simulink library "powerlib_extras"  (Simulink 6.0)
settings: Solver=ode45  SolverMode=SingleTasking  StartTime=0.0  StopTime=10.0  RelTol=1e-3
values from neighbouring files (symbols this model uses):
  Ts = get(handles.edit1,'string')    [powergui.m]
undefined symbols (not defined in the file or in its folder): Ac, Bc, Cc, Dc, Delay_discrete, dend, DiscIntNeverNeededParam, extra_sc, j, numd, test_alpha
libraries: powerlib2 x112, powerlib_extras x70, simulink_extras x25, simulink x12, powerlib_models x8
(part 1 of 9)
Description:
  | Powerlib_extras library for the Power System Blockset 2.1
settings Model: RequirementInfo=9  Creator=patrice  LastModifiedBy=batserve  ModifiedHistory=New version of the Timer block of the control library  ExtModeAutoUpdateStatusClock=off
settings DataIOCC: SignalLoggingName=logsOut
settings OptimizationCC: BooleanDataType=off
settings DebuggingCC: CheckExecutionContextPreStartOutputMsg=on  CheckExecutionContextRuntimeOutputMsg=on  SolverPrmCheckMsg=none
settings HardwareCC: TargetUnknown=on

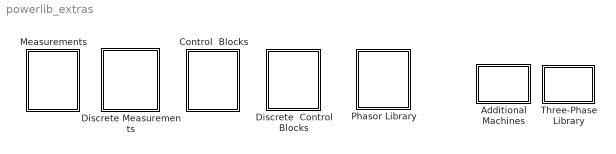
== system powerlib_extras ==
  Additional Machines : Subsystem
      mask Display: disp('obsolete\nblocks')
  Control  Blocks : Subsystem
  Discrete Measurements : Subsystem
  Discrete  Control Blocks : Subsystem
  Measurements : Subsystem
  Phasor Library : Subsystem
  Three-Phase Library : Subsystem
      mask Display: disp('Obsolete\nblocks')

== system powerlib_extras/Additional Machines ==
  DC Machine : powerlib2/Machines/DC Machine  RLa="[ 0.6  0.012]"  RLf="[ 240  120]"  Laf=1.8  J=1  Bm=0  Tf=0  w0=1  PSBOutputType=110
  Discrete DC_Machine : Subsystem  mask(Discrete DC machine){RLa=[0.5  0.01], RLf=[240  0], Laf=1.23, J=0.05, Bm=0.02, Tf=0, w0=0, PSBOutputType=110, Ts=50e-6}
      mask prompts: RLa "Armature resistance and inductance [Ra (ohms) La (H) ]"; RLf "Field resistance and inductance [Rf (ohms) Lf (H) ]"; Laf "Field-armature mutual inductance Laf (H) :"; J "Total inertia J (kg.m^2)"; Bm "Viscous friction coefficient Bm (N.m.s)"; Tf "Coulomb friction torque Tf (N.m)"; w0 "Initial speed (rad/s) :"; PSBOutputType "Output type"; Ts "Sample time (s) :"
      mask help:
      | This discrete block implements a separately excited DC machine. Access is provided  to the field connections so that the machine can be used as a shunt-connected or a series-connected  DC machine.
      |
      | Input 1 and output 1 : positive and negative armature terminals
      | Input 2 and output 2 : positive and negative field terminals
      | Input 3    : Load torque
      | Output 3 : Simulink measurement output [ w Ia If Te ]
      mask init:
      | Ra=RLa(1); La=RLa(2);
      | Rf=RLf(1); Lf=RLf(2);
      mask Help:
      | This block implements a separately excited DC machine. Access is provided  to the field connections so that the machine can be used as a shunt-connected or a series-connected  DC machine.
      | 
      | <pre>
      | The model implements the following electrical and mechanical equations:
      |     Vf  = (Rf+sLf )*If
      |     Va =   (w*Laf)*If  +  (Ra+sLaa)*Ia
      |     Te = Laf*If*Ia
      |     Te = J*dw/dt + Bm*w+ Tf + TL
      | where:
      |     Va, Vf = Armature anf field voltages (V)
      |     Ia , If = Armature anf field currents (A)
      |     w = Rotor speed (rad/s)
      |     s = Laplace derivation operator = d/dt
      |     Te = Electrical torque (N.m)
      |     TL = Load torque (N.m)
      |     Tv = Bm*w= Viscous friction torque (N.m)
      |     Tf = Coulomb friction torque (N.m)
      | 
      | Input 1 and output 1 : positive and negative armature terminals
      | Input 2 and output 2 : positive and negative field terminals
      | Input 3 : Load torque
      | Output 3 : Simulink measurement output [ w Ia If Te ]
      | 
      | In motor mode the Load torque applied on the shaft should be positive.
      | </pre>
      mask Display: plot(-80,-80,80,80,[0,9,18,24,29,30,29,24,18,9,0,-9,-18,-24,-29,-30,-29,-24,-18,-9,0],[30,29,24,18,9,0,-9,-18,-24,-29,-30,-29,-24,-18,-9,0,9,18,24,29,30],[-29,-35,-35,-29],[-8,-8,8,8],[29,35,35,29],[-8,-8,8,8],[-35,-55],[0,0],[35,55],[0,0],[-78,-50,-50,-49,-45,-39,-33,-26,-21,-18,-17,-19,-22,-22,-26,-27,-25,-22,-16,-9,-3,2,6,6,4,1,1,-3,-4,-2,2,7,14,20,26,29,30,28,24,24,21,20,21,25,31,37,44,49,50,50,50,78]*.7,[58,58,57.2,49.2,42.8,38.8,38,39.6,44.4,51.6,59.6,67.6,72.4,72.4,65.2,57.2,49.2,42.8,38.8,38,39.6,44.4,51.6,59.6,67.6,72.4,72.4,65.2,57.2,49.2,42.8,38.8,38,39.6,44.4,51.6,59.6,67.6,72.4,72.4,65.2,57.2,49.2,42.8,38.8,38,39.6,44.4,51.6,58,58,58]*.6+15 );

== system powerlib_extras/Control  Blocks ==
  note: __________ Filters__________
  note: _____________ Pulse Generators_____________
  note: __Phase-Locked Loop (PLL) Systems _______
  note: ___________________________ Miscellaneous_____________________________
  note: ___Signal Generators____
  " Synchronized 12-Pulse Generator" : Subsystem  mask(Synchronized 12-pulse generator){freq=60, pwidth=35, Double_Pulse=on}
      mask prompts: freq "Frequency of synchronisation voltages (Hz) :"; pwidth "Pulse width (degrees) :"; Double_Pulse "Double pulsing"
      mask help:
      | Use this block to fire the 12 thyristors of a 12-pulse converter. Outputs PY and PD are two vectors of 6 pulses (0-1) to be sent to the two 6-pulse half bridges connected respectively to the Wye(Y) and Delta (D) connected windings of the YYD (Delta Lagging)  converter transformer.
      |
      | Pulses are individually synchronized on the 6 commutation voltages and generated alpha degrees after the increasing zero-crossings of the commutation voltages. The D pulses are lagging the Y pulses by  30 degrees.
      |
      | When the 'Douple pulsing' option is checked, two pulses are sent to each thyristor: a 1st pulse when the aplha angle is reached, then a 2nd pulse 60 degrees later, when the next thyristor is fired.
      mask Help: web(psbhelp)
      mask Display: plot(0,0,100,100,[80 62 62 47 47 30],[40 40 60 60 40 40]-5)
  1-phase  PLL : Subsystem  mask(1-phase PLL){Par_Init=[0 60], ParK=[120 2800]}
      mask prompts: Par_Init "Initial inputs:[ Phase(degrees)   Frequency(Hz) ]"; ParK "Regulator gains [ Kp  Ki ]"
      mask help:
      | This Phase Locked Loop (PLL) system can be used  to synchronize on a variable frequency sinusoidal signal.
      |
      | Input 1: Normalized input signal V(pu)
      |
      | Output 1:  Measured frequency (Hz) = w/(2pi)
      | Output 2:  Ramp w.t  varying between  0 and 2*pi, synchronized on the zero-crossing (rising) of  the input signal
      | Output 3: Vector [sin(wt) cos(wt)]
      mask init:
      | Kp=ParK(1);
      | Ki=ParK(2);
      | Phase_Init=Par_Init(1);
      | Finit=Par_Init(2);
  1st-Order  Filter : Subsystem  mask(First-Order Filter){FilterType=Lowpass, Tc=12e-3, Initialize=off, Vac_Init=[0.8 -25 60], Vdc_Init=-0.4, PlotResponse=off, param1=[1 500 1]}
      mask prompts: FilterType "Filter Type:"; Tc "Time constant (s):"; Initialize "Initialize filter states"; Vac_Init "AC initial input: [ Mag  Phase(degrees)  Freq(Hz) ]"; Vdc_Init "DC Initial input:"; PlotResponse "Plot filter response"; param1 "Frequency range(Hz) : [Start  End  Inc.]"
      mask init:
      | switch FilterType
      | case 1, % Lowpass
      |        X=[0 1 2 3 4];
      |        Y=[-2 -2 -3 -4 -4];
      |        numc=1;
      |        denc=[Tc 1];
      |  case 2,   % Highpass
      |        X=[0 1 2 3 4];
      |        Y=[-4 -4 -3 -2 -2];
      |         numc=[1 0];
      |         denc=[1 1/Tc];
      | end
      | %
      | [Ac,Bc,Cc,Dc]=tf2ss(numc,denc);
      | %
      | %
      | if Initialize==1  % Compute initial conditions on states
      | u1=Vac_Init(1)*exp(j*Vac_Init(2)*pi/180);
      | u2=Vdc_Init*exp(j*90*pi/180);
      | u=u1+u2;
      | u0=imag(u); % input at  t=0;
      | I=eye(size(Ac));
      | sI1=I*j*(2*pi*Vac_Init(3));
      | sI2=I*j*0;
      | x=inv(sI1-Ac)*Bc*u1 + inv(sI2-Ac)*Bc*u2;
      | x0c=imag(x);
      | else
      | x0c=0;
      | end
      | %
      | if PlotResponse==1 % Plot frequency and step response
      | t=[0:Tc/1000:7*Tc];
      | f=param1(1):param1(3):param1(2);
      | w=2*pi*f;
      | switch FilterType
      | 	case 1, % Lowpass
      | 		Ystep=1 - exp(-t/Tc);
      | 		RepFreq=1./(1+Tc*j.*w);
      | 	case 2,   % Highpass
      | 		Ystep=exp(-t/Tc);
      | 		RepFreq=1./(1 + (1./(Tc*j.*w)));
      | end
      | %
      | Mag=abs(RepFreq);
      | Pha=angle(RepFreq)*180/pi;
      | %
      | figure(1)
      | subplot(2,1,1)
      | plot(f,Mag)
      | grid
      | title('Bode Diagram')
      | ylabel('Magnitude')
      | subplot(2,1,2)
      | plot(f,Pha)
      | ylabel('Phase (deg)')
      | xlabel('Frequency (Hz)')
      | grid
      | figure(2)
      | plot(t,Ystep)
      | grid
      | ylabel('Amplitude')
      | xlabel('Time (s)')
      | title('Step Response')
      | end
      mask StyleString: popup(Lowpass|Highpass),edit,checkbox,edit,edit,checkbox,edit
      mask CallbackString: ||parametres=get_param(gcb,'MaskValues');p3=parametres{3};p6=parametres{6};if strcmp(p3,'on');param4='on';param5='on';else;param4='off';param5='off';end;if strcmp(p6,'on');param7='on';else;param7='off';end;visible={'on','on','on',param4,param5,'on',param7};set_param(gcb,'MaskVisibilities',visible)|||parametres=get_param(gcb,'MaskValues');p3=parametres{3};p6=parametres{6};if strcmp(p3,'on');param4='on';param5='on';else;param4='off';param5='off';end;if strcmp(p6,'on');param7='on';else;param7='off';end;visible={'on','on','on',param4,param5,'on',param7};set_param(gcb,'MaskVisibilities',visible)|
      mask Display: plot(X,Y);
  2nd-Order Filter : Subsystem  mask(2nd-Order Filter){FilterType=Lowpass, Fo=200, Zeta=0.707, Initialize=off, Vac_Init=[1 45 60], Vdc_Init=-0.5, PlotResponse=off, param1=[1 500 1]}
      mask prompts: FilterType "Filter Type:"; Fo "Cut-off frequency (Hz):"; Zeta "Damping factor Zeta ( Q = 1 / (2*Zeta) ):"; Initialize "Initialize filter states"; Vac_Init "AC initial input: [ Mag  Phase(degrees)  Freq(Hz) ]"; Vdc_Init "DC Initial input:"; PlotResponse "Plot filter response"; param1 "Frequency range(Hz) : [Start  End  Inc.]"
      mask init:
      | Wo=2*pi*Fo;
      | str=sprintf(' Fo=%iHz\n\n',Fo);
      | switch FilterType
      | case 1, % Lowpass
      |        X=[0 1 2 3 4];
      |        Y=[-2 -2 -3 -4 -4];
      |        n2=0;n1=0;n0=Wo*Wo;
      |        d2=1;d1=2*Zeta*Wo;d0=Wo*Wo;
      |  case 2,   % Highpass
      |        X=[0 1 2 3 4];
      |        Y=[-4 -4 -3 -2 -2];
      |        n2=1;n1=0;n0=0;
      |        d2=1;d1=2*Zeta*Wo;d0=Wo*Wo;
      |     case 3,   % Bandpass
      |        X=[0 1 2 3 4 5 ];
      |        Y=[-3 -3 -2 -2 -3 -3];
      |        n2=0;n1=2*Zeta*Wo;n0=0;
      |        d2=1;d1=2*Zeta*Wo;d0=Wo*Wo;
      |     case 4,  %Bandstop (Notch)
      |        X=[0 1 2 3 4 5 ];
      |        Y=[-2 -2 -3 -3 -2 -2];
      |        n2=1;n1=0;n0=Wo*Wo;
      |        d2=1;d1=2*Zeta*Wo;d0=Wo*Wo;
      |     end
      | %
      | numc=[n2 n1 n0];
      | denc=[d2 d1 d0];
      | [Ac,Bc,Cc,Dc]=tf2ss(numc,denc);
      | %
      | if Initialize==1  % Compute initial conditions on states
      | u1=Vac_Init(1)*exp(j*Vac_Init(2)*pi/180);
      | u2=Vdc_Init*exp(j*90*pi/180);
      | u=u1+u2;
      | u0=imag(u); % input at  t=0;
      | I=eye(size(Ac));
      | sI1=I*j*(2*pi*Vac_Init(3));
      | sI2=I*j*0;
      | x=inv(sI1-Ac)*Bc*u1 + inv(sI2-Ac)*Bc*u2;
      | x0c=imag(x);
      | else
      | x0c=0;
      | end
      | %
      | if PlotResponse==1 % Plot frequency and step response
      | if Zeta==1
      | 	z=1+1e-12;
      | else
      | 	z=Zeta;
      | end
      | wn=Wo;
      | t=[0:1/(z*wn)/1000:7/(z*wn)];
      | f=param1(1):param1(3):param1(2);
      | w=2*pi*f;
      | switch FilterType
      | 	case 1, % Lowpass
      | 		Ystep=wn^2*(1/wn^2+1/(4*z^2*wn^2-4*wn^2)^(1/2)*(1/(-z*wn+1/2*(4*z^2*wn^2-4*wn^2)^(1/2))*exp((-z*wn+1/2*(4*z^2*wn^2-4*wn^2)^(1/2))*t)-1/(-z*wn-1/2*(4*z^2*wn^2-4*wn^2)^(1/2))*exp((-z*wn-1/2*(4*z^2*wn^2-4*wn^2)^(1/2))*t)));
      | 		numFreq=wn^2;
      | 	case 2,   % Highpass
      | 		Ystep=-exp(-z*wn*t)/(z-1)/(z+1).*cos((-wn^2*(z-1)*(z+1))^(1/2)*t)+exp(-z*wn*t)/(z-1)/(z+1)*z^2.*cos((-wn^2*(z-1)*(z+1))^(1/2)*t)+z/wn*exp(-z*wn*t)/(z-1)/(z+1)*(wn^2-z^2*wn^2)^(1/2).*sin((-wn^2*(z-1)*(z+1))^(1/2)*t);
      | 		numFreq=-w.^2;
      | 	case 3,   % Bandpass
      | 		Ystep=2*z*wn/(4*z^2*wn^2-4*wn^2)^(1/2)*(exp((-z*wn+1/2*(4*z^2*wn^2-4*wn^2)^(1/2))*t)-exp((-z*wn-1/2*(4*z^2*wn^2-4*wn^2)^(1/2))*t));
      | 		numFreq=2*Zeta*wn.*w*j;
      | 	case 4,  %Bandstop (Notch)
      | 		Ystep=1+2*z/wn*exp(-z*wn*t)/(z-1)/(z+1)*(wn^2-z^2*wn^2)^(1/2).*sin((-wn^2*(z-1)*(z+1))^(1/2)*t);	
      | 		numFreq=wn^2-w.^2;
      | end
      | %
      | denFreq=(wn^2-w.^2) + 2*Zeta*wn*j.*w;
      | RepFreq=numFreq./denFreq;
      | Mag=abs(RepFreq);
      | Pha=angle(RepFreq)*180/pi;
      | %
      | figure(1)
      | subplot(2,1,1)
      | plot(f,Mag)
      | grid
      | title('Bode Diagram')
      | ylabel('Magnitude')
      | subplot(2,1,2)
      | plot(f,Pha)
      | ylabel('Phase (deg)')
      | xlabel('Frequency (Hz)')
      | grid
      | figure(2)
      | plot(t,real(Ystep))
      | grid
      | ylabel('Amplitude')
      | xlabel('Time (s)')
      | title('Step Response')
      | end
      mask StyleString: popup(Lowpass|Highpass|Bandpass|Bandstop (Notch)),edit,edit,checkbox,edit,edit,checkbox,edit
      mask CallbackString: |||parametres=get_param(gcb,'MaskValues');p4=parametres{4};p7=parametres{7};if strcmp(p4,'on');param5='on';param6='on';else;param5='off';param6='off';end;if strcmp(p7,'on');param8='on';else;param8='off';end;visible={'on','on','on','on',param5,param6,'on',param8};set_param(gcb,'MaskVisibilities',visible)|||parametres=get_param(gcb,'MaskValues');p4=parametres{4};p7=parametres{7};if strcmp(p4,'on');param5='on';param6='on';else;param5='off';param6='off';end;if strcmp(p7,'on');param8='on';else;param8='off';end;visible={'on','on','on','on',param5,param6,'on',param8};set_param(gcb,'MaskVisibilities',visible)|
      mask Display:
      | plot(X,Y);
      | disp(str);
  3-phase  Programmable Source : Subsystem  mask(3-phase Programmable Source){Par_Vps=[1.0 -20  60], VariationEntity=Amplitude, VariationType=Step, VariationStep=-0.5, VariationRate=10, VariationMag=0.3, VariationFreq=2, Par_Timing_Variation=[0.1 1.2], SinglePhase=off, Yampli=[1 0.8 1.2 1.0], Xtime=[0 0.1 0.15 0.2], HarmonicGeneration=off, Par_HarmoA=[3 0.2 -25 0], Par_HarmoB=[2 0.15 35 2], Par_Timing_Harmo=[0.05  3]}
      mask prompts: Par_Vps "Positive-sequence: [ Amplitude  Phase(degrees)   Freq. (Hz) ]"; VariationEntity "Time variation of:"; VariationType "Type of variation:"; VariationStep "Step magnitude:"; VariationRate "Rate of change (value/s):"; VariationMag "Amplitude of the modulation:"; VariationFreq "Frequency of the modulation(Hz):"; Par_Timing_Variation "Variation timing (s) : [ Start   End ]"; SinglePhase "1-phase only"; Yampli "Amplitude values:"; Xtime "Time values:"; HarmonicGeneration "Harmonic generation:"; Par_HarmoA "A:  [ Order(n)   Amplitude  Phase(degrees)  Seq(0, 1 or 2) ]"; Par_HarmoB "B:  [ Order(n)   Amplitude  Phase(degrees)  Seq(0, 1 or 2) ]"; Par_Timing_Harmo "Harmonic timing (s) : [ Start   End ]"
      mask help: Use this block to generate a set of three-phase sinusoidal voltages or currents a, b and c. Time variation for the amplitude, phase and frequency of the fundamental can be pre-programmed. In addition, two harmonics can be surimposed on the fundamental.
      mask init:
      | Mag_Vps=Par_Vps(1);
      | Phase_Vps=Par_Vps(2);
      | Freq_Vps=Par_Vps(3);
      | 
      | Ton_Variation=Par_Timing_Variation(1);
      | Toff_Variation=Par_Timing_Variation(2);
      | n_HarmoA=Par_HarmoA(1);
      | Mag_HarmoA=Par_HarmoA(2);
      | Phase_HarmoA=Par_HarmoA(3);
      | Seq_HarmoA=Par_HarmoA(4);
      | if n_HarmoA==0
      |     Phase_HarmoA=90;
      |     Seq_HarmoA=0;
      | end
      | n_HarmoB=Par_HarmoB(1);
      | Mag_HarmoB=Par_HarmoB(2);
      | Phase_HarmoB=Par_HarmoB(3);
      | Seq_HarmoB=Par_HarmoB(4);
      | if n_HarmoB==0
      |     Phase_HarmoB=90;
      |     Seq_HarmoB=0;
      | end
      | Ton_Harmo=Par_Timing_Harmo(1);
      | Toff_Harmo=Par_Timing_Harmo(2);
      | 
      | if Xtime(1)~=0,
      | Xtime=[0 Xtime];
      | Yampli=[0 Yampli];
      | end
      | n=length(Xtime); vec_dt= [Xtime,0] - [0,Xtime] ; vec_dt=vec_dt(2:n);
      mask StyleString: edit,popup(None|Amplitude|Phase|Frequency),popup(Step|Ramp|Modulation|Table of time-amplitude pairs),edit,edit,edit,edit,edit,checkbox,edit,edit,checkbox,edit,edit,edit
      mask CallbackString: |parametres=get_param(gcb,'MaskValues');p2=parametres{2};p3=parametres{3};p12=parametres{12};if strcmp(p3,'Step');param4='on';param5='off';param6='off';param7='off';param8='on';param9='off';param10='off';param11='off';elseif strcmp(p3,'Ramp');param4='off';param5='on';param6='off';param7='off';param8='on';param9='off';param10='off';param11='off';elseif strcmp(p3,'Modulation');param4='off';param5='off';param6='on';param7='on';param8='on';param9='off';param10='off';param11='off';else;param4='off';param5='off';param6='off';param7='off';param8='off';param9='on';param10='on';param11='on';end;if strcmp(p2,'None');param3='off';param4='off';param5='off';param6='off';param7='off';param8='off';param9='off';param10='off';param11='off';else;param3='on';end;if strcmp(p12,'on');param13='on';param14='on';param15='on';else;param13='off';param14='off';param15='off';end;visible={'on','on',param3,param4,param5,param6,param7,param8,param9,param10,param11,'on',param13,param14,param15};set_param(gcb,'MaskVisibilities',visible)|parametres=get_param(gcb,'MaskValues');p2=parametres{2};p3=parametres{3};p12=parametres{12};if strcmp(p3,'Step');param4='on';param5='off';param6='off';param7='off';param8='on';param9='off';param10='off';param11='off';elseif strcmp(p3,'Ramp');param4='off';param5='on';param6='off';param7='off';param8='on';param9='off';param10='off';param11='off';elseif strcmp(p3,'Modulation');param4='off';param5='off';param6='on';param7='on';param8='on';param9='off';param10='off';param11='off';else;param4='off';param5='off';param6='off';param7='off';param8='off';param9='on';param10='on';param11='on';end;if strcmp(p2,'None');param3='off';param4='off';param5='off';param6='off';param7='off';param8='off';param9='off';param10='off';param11='off';else;param3='on';end;if strcmp(p12,'on');param13='on';param14='on';param15='on';else;param13='off';param14='off';param15='off';end;visible={'on','on',param3,param4,param5,param6,param7,param8,param9,param10,param11,'on',param13,param14,param15};set_param(gcb,'MaskVisibilities',visible)|||||||||parametres=get_param(gcb,'MaskValues');p2=parametres{2};p3=parametres{3};p12=parametres{12};if strcmp(p3,'Step');param4='on';param5='off';param6='off';param7='off';param8='on';param9='off';param10='off';param11='off';elseif strcmp(p3,'Ramp');param4='off';param5='on';param6='off';param7='off';param8='on';param9='off';param10='off';param11='off';elseif strcmp(p3,'Modulation');param4='off';param5='off';param6='on';param7='on';param8='on';param9='off';param10='off';param11='off';else;param4='off';param5='off';param6='off';param7='off';param8='off';param9='on';param10='on';param11='on';end;if strcmp(p2,'None');param3='off';param4='off';param5='off';param6='off';param7='off';param8='off';param9='off';param10='off';param11='off';else;param3='on';end;if strcmp(p12,'on');param13='on';param14='on';param15='on';else;param13='off';param14='off';param15='off';end;visible={'on','on',param3,param4,param5,param6,param7,param8,param9,param10,param11,'on',param13,param14,param15};set_param(gcb,'MaskVisibilities',visible)|||
  3-phase PLL : Subsystem  mask(3-phase PLL){Par_Init=[0 60], ParK=[60 1400]}
      mask prompts: Par_Init "Initial inputs:[ Phase(degrees)   Frequency(Hz) ]"; ParK "Regulator gains [ Kp  Ki ]"
      mask help:
      | This Phase Locked Loop (PLL) system can be used  to synchronize on a set of variable frequency, three-phase sinusoidal signals.
      |
      | Input 1: Vector containing the normalized
      |              three-phase signals [Va Vb Vc]
      | Output 1:  Measured frequency (Hz) = w/(2pi)
      | Output 2:  Ramp w.t   varying between  0 and 2*pi,
      | synchronized on zero crossings of the fundamental (positive-sequence) of phase A.
      | Output 3: Vector [sin(wt) cos(wt)]
      mask init:
      | Kp=ParK(1);
      | Ki=ParK(2);
      | Phase_Init=Par_Init(1);
      | Finit=Par_Init(2);
  Bistable : Subsystem  AncestorBlock=|  mask(Bistable Flip-Flop (Priority to Set or Reset)){priority=Set, ic=0}
      | powerlib_extras/Discrete 
      | Control Blocks/Discrete
      | Bistable
      mask prompts: priority "Priority to input:"; ic "Initial Q output (0/1):"
      mask help:
      | SR Flip-Flop block, with priority given either  to the Set  (S) or Reset  (R) input.
      |
      | Priority to Set: If inputs S (set) and R (reset) are TRUE (1) simultaneously, the output Q is set to TRUE (1).
      |
      | Priority to Reset: If inputs S (set) and R (reset) are TRUE (1) simultaneously, the output Q is reset to FALSE (0).
      |
      | The  Q! output  is the complement of the Q output.
      | The initial value of the Q output  is specified by the parameter "Initial Q output".
      mask init:
      | if (priority==1)   % RESET
      |  str1 = '[R]';
      |  str2 = 'S';
      | else
      | str1= 'R';
      | str2 = '[S]';
      | end
      mask StyleString: popup(Reset|Set),edit
      mask Display:
      | plot(0,0,100,100);
      | text(5,25,str1);
      | text(5,75,str2);
      | text(72,25,'!Q');
      | text(78,75,'Q');
  Edge Detector : Subsystem  mask(Edge Detector){model=Rising, ic=0}
      mask prompts: model "Edge:"; ic "Input at t = -eps:"
      mask help:
      | This block compares its present input to its previous input.
      |
      | If the input  is a logic signal (TRUE (1) or FALSE (0), the output is a one-step boolean signal TRUE  when  the specified edge (Rising, Falling or Either)  is detected.
      |
      | This block can also be used to detect the slope polarity of a continuous signal. For example, if the specified edge is  "Rising", the output is TRUE as long as the slope of the input signal is positive.
      |
      | The input value at time preceeding t=0 is specified by the parameter "Input at t=-eps"
      mask init:
      | if model~=3,
      | 	x1 = (model -1)*20;
      |     x2 = (model -1)*60;
      | 	X1=[5,20,20,35]+25; Y1=[20+x2,20+x2,80-x2,80-x2];
      | 	X2=[5,20,35]+25;    Y2=[40+x1,60-x1,40+x1];
      | 	X3=[];X4=[];Y3=[];Y4=[];
      | else
      | 	x1 = 20;
      | 	x2 = 60;
      | 	X1=[5,20,20,35]+8; Y1=[20,20,80,80];
      | 	X2=[5,20,35]+8;    Y2=[40,60,40];
      | 	X3=[5,20,20,35]+53; Y3=[20+x2,20+x2,80-x2,80-x2];
      | 	X4=[5,20,35]+53;    Y4=[40+x1,60-x1,40+x1];
      | end
      mask StyleString: popup(Rising|Falling|Either),edit
      mask Display: plot(0,0,100,100, X1,Y1,X2,Y2,X3,Y3,X4,Y4);
  Monostable : Subsystem  mask(Monostable Flip-Flop){EdgeDetect=Either, t_mono=0.015, ic=0}
      mask prompts: EdgeDetect "Edge detection"; t_mono "Pulse duration (s):"; ic "Input at t = -eps:"
      mask help:
      | After being triggered  by the specified edge (Rising, Falling or Either), this block outputs a pulse (TRUE signal) for the time specified by parameter "Pulse duration".
      | If the specified edge is detected while the output is TRUE, the monostable is not retriggered
      |
      | The input value (0/1) at time preceeding t = 0 is specified by the parameter "input at t = -eps".
      mask init:
      | str=sprintf('%g %c',t_mono,'s');
      | if (EdgeDetect ~=3)
      |     x1 = (EdgeDetect -1)*10;
      |     x2 = (EdgeDetect -1)*30;
      | 	X1=[15-8,25,25,35+8]+0; Y1=[65+x2,65+x2,95-x2,95-x2];
      | 	X2=[15,25,35]+0;   Y2=[75+x1,85-x1,75+x1];
      | 	X3=[];X4=[];Y3=[];Y4=[];	
      | else
      | 	x1 = 10;
      | 	x2 = 30;
      | 	X1=[15,25,25,35]-14;  Y1=[65,65,95,95];
      | 	X2=[15,25,35]-14;    Y2=[75,85,75];
      | 	X3=[15,25,25,35]+14; Y3=[65+x2,65+x2,95-x2,95-x2];
      | 	X4=[15,25,35]+14;   Y4=[75+x1,85-x1,75+x1];
      | end
      mask StyleString: popup(Rising|Falling|Either),edit,edit
      mask Display:
      | plot(0,0,100,100,[100 75 75 25 25 0],[25 25 50 50 25 25]-0,X1,Y1,X2,Y2,X3,Y3,X4,Y4);
      | text(45,37,'T');
      | text(15,15,str);
  On/Off Delay : Subsystem  AncestorBlock=|  mask(On/Off Delay ){type_delay=On delay, delay=0.01, ic=0}
      | powerlib_extras/Discrete 
      | Control Blocks/Discrete
      | On//Off Delay
      mask prompts: type_delay "Type:"; delay "Time delay:"; ic "Input at t = -eps (0/1):"
      mask help:
      | Apply a delay on the input signal when the input changes to TRUE (1) or FALSE (0).
      |
      | On delay: When the input becomes TRUE, the output becomes TRUE after the specified time delay as long as the input is still TRUE. If the input becomes FALSE before the time delay has expired , the output stays FALSE.
      |
      | Off delay: When the input becomes FALSE, the output becomes FALSE after the specified time delay as long as the input is still FALSE. If the input becomes TRUE before the time delay has expired , the output stays TRUE.
      |
      | The input value (0/1) at time preceeding t=0 is specified by the parameter "input at t = -eps".
      mask init:
      | str=sprintf('%g %c',delay,'s');
      mask StyleString: popup(On delay|Off delay),edit,edit
      mask Display:
      | plot(0,0,100,100,[10,10,10,90,90,90],[60,40,50,50,40,60]);
      | text(25+(type_delay-1)*50,80,'t');
      | text(15,20,str);
  PWM Generator : Subsystem  mask(PWM Generator){GeneratorMode=Double 3-arm  bridges (12 pulses), Fc=1080, Internal=on, mIndex=0.4, Freq=60, Phase=0}
      mask prompts: GeneratorMode "Generator Mode"; Fc "Carrier frequency (Hz):"; Internal "Internal generation of modulating signal(s)"; mIndex "Modulation index  (0<m<1) :"; Freq "Frequency of output voltage (Hz)"; Phase "Phase of output voltage (degrees)"
      mask help:
      | This block generates pulses for carrier-based PWM (Pulse Width Modulation), self-commutated IGBTs,GTOs or FETs bridges.
      |
      | Depending on the number of bridge arms selected in the "Generator Mode" parameter, the block can be used either for single-phase or three-phase PWM control.
      |
      | Press Help for details on input(s) and outputs.
      |
      | See psb1phPWM and psb3phPWM demos respectively  for application examples of single-phase and three-phase inverters using the discrete version of this block.
      mask init:
      | if Freq==0
      |     Phase=90;
      | end
      | switch GeneratorMode
      | case 1,
      |     Internal_Phase=0;
      |    Signal_PortWidth=1;
      |    Select1_Elements=[1 2];
      |    Select1_PortWidth=2;
      |    Select3_Elements=[1 2];
      |    Select3_PortWidth=4;
      | case 2,
      |     Internal_Phase=0;
      |     Signal_PortWidth=1;
      |     Select1_Elements=[1 2];
      |     Select1_PortWidth=2;
      |     Select3_Elements=[1 2 3 4];
      |     Select3_PortWidth=4;
      | case 3,
      |     Internal_Phase=[0 -2*pi/3 2*pi/3];
      |     Signal_PortWidth=3;
      |     Select1_Elements=[1 4 2 5 3 6];
      |     Select1_PortWidth=6;
      |    Select3_Elements=[1 2 3 4 5 6];
      |    Select3_PortWidth=12;
      | case 4,
      |     Internal_Phase=[0 -2*pi/3 2*pi/3];
      |     Signal_PortWidth=3;
      |     Select1_Elements=[1 4 2 5 3 6];
      |     Select1_PortWidth=6;
      |    Select3_Elements=[1 2 3 4 5 6 7 8 9 10 11 12];
      |    Select3_PortWidth=12;
      | end
      mask Help: web(psbhelp)
      mask StyleString: popup(1-arm  bridge (2 pulses)|2-arm  bridge (4 pulses)|3-arm  bridge (6 pulses)|Double 3-arm  bridges (12 pulses)),edit,checkbox,edit,edit,edit
      mask CallbackString: ||p3=get_param(gcb,'Internal');if strcmp(p3,'on');visible={'on','on','on','on','on','on'};else;visible={'on','on','on','off','off','off'};end;set_param(gcb,'MaskVisibilities',visible)|||
  Sample & Hold : Subsystem  mask(Sample & Hold ){ic=0}
      mask prompts: ic "Initial condition:"
      mask help: The output follows input 1 (In) as long as input 2 (S) is TRUE (1) . The output is held when input 2 becomes FALSE (0). The output initial value is specified by the parameter "Initial condition".
      mask Display: disp('S/H')
  Synchronized 6-Pulse Generator : Subsystem  mask(Synchronized 6-pulse generator){freq=60, pwidth=10, Double_Pulse=off}
      mask prompts: freq "Frequency of synchronisation voltages (Hz) :"; pwidth "Pulse width (degrees) :"; Double_Pulse "Double pulsing"
      mask help: Use this block to fire the 6 thyristors of a 6-pulse converter. The output is a vector of 6 pulses (0-1) individually synchronized on the 6 commutation voltages. Pulses are generated alpha degrees after the increasing zero-crossings of the commutation voltages.
      mask Help: web(psbhelp)
      mask Display: plot(0,0,100,100,[80 62 62 47 47 30],[40 40 60 60 40 40]-5)
  Timer : Subsystem  mask(Timer){t=[ 0  1  3  3.5  ], e=[1  -1  2.5  0   ]}
      mask prompts: t "Time (s):"; e "Amplitude:"
      mask help:
      | Generates a signal changing at specified times.
      |
      | If a signal value is not specified at time zero, the output is kept at 0 until the first specified transition time.
      mask init:
      | tt=t;
      | sv=e;
      | %
      | if length(sv) ~= length(tt),
      |    h=errordlg(' The vectors specifying the time and amplitude pairs must have the same length ' , 'Parameter error');
      | end
      | if tt(1)~=0,
      |    tt=[0 tt];
      |    sv=[~sv(1) sv];
      | end
      | n=length(tt);
      | vec_dt=[tt,0]-[0,tt] ;
      | vec_dt=vec_dt(2:n);
      | if any(vec_dt<=0)
      |    h=errordlg(' All transition times must be in increasing order' , 'Parameter error');
      | end
      | tv=[-1,tt(1),reshape(repmat(reshape(tt(2:end),1,length(tt)-1),2,1),1,2*length(tt)-2),tt(end)+1];
      | %sv=(sv(:)'~=0);
      | opv=[sv(1),reshape(repmat(sv(1:end-1),2,1),1,2*length(sv)-2),sv(end),sv(end)];
      mask Help: web(psbhelp)
      mask Display: plot( tv(2:end-1), opv(2:end-1) )

== system powerlib_extras/Discrete Measurements ==
  note: ____ Single-Phase Measurements _________________________________________________________________
  note: ____ Three-Phase Measurements __________________________________________________________________
  note: ____ Power Measurements ________________________________________________________________________
  note: ____ Miscellaneous __________________
  3-phase  Instantaneous  Active & Reactive Power : powerlib_extras/Measurements/3-phase  Instantaneous  Active & Reactive Power
  Discrete PLL-Driven  Fundamental Value : Subsystem  mask(Discrete PLL-Driven Fundamental Value){Finit=60, Fmin=45, Par_Init=[1 30], Ts=50e-6}
      mask prompts: Finit "Initial frequency (Hz):"; Fmin "Minimum frequency (Hz):"; Par_Init "Initial input: [ Mag  Phase-relative-to-PLL(degrees) ]"; Ts "Sample time:"
      mask help:
      | This discrete block computes the fundamental value of the input signal (port In) over a running window of one cycle of a specified fundamental frequency (port Freq). Input port "Sin_Cos" (a two-dimension signal) provides the reference frame required for the computation..
      |  First and second outputs return respectively the magnitude and phase (in degrees relative to the PLL phase) of the fundamental.
      |
      | For the first cycle of simulation, the ouputs are held constant to the values specified by the parameter "Initial input". The value of the parameter "Minimum frequency" is used to determine the buffer size of the "Variable Transport Delay" block found inside this subsystem.
      mask init:
      | Real_Init=Par_Init(1)*cos(pi/180*Par_Init(2));
      | Imag_Init=Par_Init(1)*sin(pi/180*Par_Init(2));
  Discrete Variable Frequency Mean value : Subsystem  mask(Discrete Variable-Frequency Mean Value){Finit=60, Fmin=45, Vinit=0, Ts=50e-6}
      mask prompts: Finit "Initial frequency (Hz):"; Fmin "Minimum frequency (Hz):"; Vinit "Initial input (DC component):"; Ts "Sample time:"
      mask help:
      | This discrete block computes the mean value of the input signal (port In) over a running window of one cycle of a specified frequency (port Freq).
      |
      | For the first cycle of simulation (specified by the parameter "Initial frequency"), the ouput is held to the value of the  "Initial input" parameter.
      |
      | The value of the parameter "Minimum frequency" is used to determine the buffer size of the "Variable Transport Delay" block found inside this subsystem.
      mask init:
      | MaxDelay=1/Fmin+Ts;
  Discrete  Active  & Reactive  Power : Subsystem  mask(Discrete Active & Reactive Power ){Freq=60, Par_Vinit=[0 0], Par_Iinit=[0 0], Ts=50e-6}
      mask prompts: Freq "Fundamental frequency (Hz):"; Par_Vinit "Voltage initial input: [ Mag  Phase(degrees) ]"; Par_Iinit "Current initial input: [ Mag  Phase(degrees) ]"; Ts "Sample time:"
      mask help:
      | This discrete block measures the active power P and reactive power Q, ,at fundamental frequency  of  a periodic set of voltage and current which may contain harmonics. P and Q are calculated by evaluating the fundamental values of the input voltage and current with a running window over one cycle of the fundamental frequency.
      |
      | input 1: Instantaneous voltage (V)
      | input 2: Instantaneous current (A)
      | Output 1: Vector of the fundamental values (Magnitude) of the voltage & current
      | Output 2: PQ measurement vector [P(W) Q (var)] evaluated at the fundamental frequency.
      | Sign convention: Current flowing into an RL circuit will
      | produce  positive active and reactive powers.
      |
      | For the first cycle of simulation, the ouputs are held constant using the values specified by the parameters "Initial input".
  Discrete  Fourier : Subsystem  mask(Discrete Fourier){Freq=60, n=1, Par_Init=[0 0], Ts=50e-6}
      mask prompts: Freq "Fundamental frequency (Hz):"; n "Harmonic n (0=DC; 1=fundamental; 2=2nd harm;  ...):"; Par_Init "Initial input: [ Mag  Phase(degrees) ]"; Ts "Sample time:"
      mask help:
      | This block computes the fundamental value of the input signal over a running window of one cycle of the specified fundamental frequency. First and second outputs return respectively the magnitude and phase (degrees) of the fundamental.
      | For the first cycle of simulation, the ouputs are held constant to the value specified by the parameter "Initial input".
      mask init:
      | k=2-(n==0);
      | SamplesPerCycle=1/Freq/Ts;
      | RoundSamplesPerCycle=round(SamplesPerCycle);
      | Delay=RoundSamplesPerCycle*Ts - Ts/2;
      | Correction=SamplesPerCycle/RoundSamplesPerCycle - 1;
      | Real_Init=Par_Init(1)*cos(pi/180*Par_Init(2));
      | Imag_Init=Par_Init(1)*sin(pi/180*Par_Init(2));
  Discrete  Mean value : Subsystem  mask(Discrete Mean value){Freq=60, Vinit=0, Ts=50e-6}
      mask prompts: Freq "Fundamental frequency (Hz):"; Vinit "Initial input (DC component):"; Ts "Sample time:"
      mask help:
      | This block computes the mean value of the input signal over a running window of one cycle of the specified fundamental frequency.
      | For the first cycle of simulation, the ouput is held constant to the value specified by the parameter "Initial input".
      mask init:
      | SamplesPerCycle=1/Freq/Ts;
      | RoundSamplesPerCycle=ceil(SamplesPerCycle);
      | Delay=RoundSamplesPerCycle*Ts;
      | Corr1=(SamplesPerCycle-RoundSamplesPerCycle)/2;
      | Corr2=(SamplesPerCycle-RoundSamplesPerCycle)/SamplesPerCycle;
      | K1=Corr1*Corr2;
      | K2=Corr2 + Corr1*Corr2;
  Discrete  RMS value : Subsystem  mask(Discrete RMS value){Freq=60, Mag_Init=0, Ts=50e-6}
      mask prompts: Freq "Fundamental frequency (Hz):"; Mag_Init "Initial magnitude of input:"; Ts "Sample time:"
      mask help:
      | This discrete block measures the root mean square value of instantaneous current or voltage signal connected to the input of the block. The RMS value is calculated over a running window of one cycle of the specified fundamental frequency.
      | For the first cycle of simulation, the ouput is held constant to the RMS value of the specified magnitude of initial input.
  Discrete  Total  Harmonic Distorsion : Subsystem  mask(Discret Total Harmonic Distortion ){Freq=60, Ts=50e-6}
      mask prompts: Freq "Fundamental frequency (Hz):"; Ts "Sample time:"
      mask help:
      | This discrete block measures the total harmonic distortion  (THD ) of a periodic instantaneous voltage or current connected to the input.
      | The THD is defined as:
      |
      |                   THD = Uh/U1
      | where:
      |    Uh = rms value of the harmonics
      |          = sqrt(U2^2 + U3^2 + ....+ Un^2 +...)
      |    U1 = rms value of the fundamental component
  Discrete 3-phase PLL-Driven Positive-Sequence Fundamental Value : Subsystem  mask(Discrete 3-phase PLL-Driven Positive-Sequence Fundamental Value){Finit=60, Fmin=45, Par_Init=[0 0], Ts=50e-6}
      mask prompts: Finit "Initial frequency (Hz):"; Fmin "Minimum frequency (Hz):"; Par_Init "Initial input (positive component): [ Mag  Phase-relative-to-PLL(degrees) ]"; Ts "Sample time:"
      mask help:
      | For a supplied fundamental frequency (port Freq), this discrete block computes  the positive-sequence component (Magnitude and Phase)  of a set of three balanced or unbalanced signals (port abc) which may contain harmonics.
      |  Input port "Sin_Cos" (a two-dimension signal) provides the reference frame required for the computation..
      |  First and second outputs return respectively the magnitude and phase (in degrees relative to the PLL phase)) of the fundamental.
      | For the first cycle of simulation, the ouputs are held constant to the values specified by the parameter "Initial input".
      | constant to the values specified by the parameter "Initial input". The value of the parameter "Minimum frequency" is used to determine the buffer size of the "Variable Transport Delay" block found inside this subsystem.
      mask init:
      | Real_Init=Par_Init(1)*cos(pi/180*Par_Init(2));
      | Imag_Init=Par_Init(1)*sin(pi/180*Par_Init(2));
  Discrete 3-phase PLL-Driven  Positive-Sequence Active & Reactive Power : Subsystem  mask(Discrete 3-phase PLL-Driven Positive-Sequence Active & Reactive Power ){Finit=60, Fmin=45, Par_Vinit=[1 30], Par_Iinit=[0.5 -10], Ts=50e-6}
      mask prompts: Finit "Initial frequency (Hz):"; Fmin "Minimum frequency (Hz):"; Par_Vinit "Voltage initial input: [ Mag  Phase(Degrees) ]"; Par_Iinit "Current initial input: [ Mag  Phase(Degrees) ]"; Ts "Sample time:"
      mask help:
      | This discrete block measures the 3-phase active power P and reactive power Q  associated with a periodic set of 3-phase voltages and currents which may contain harmonics. P and Q are calculated by evaluating the fundamental values (positive-sequence) of the input voltages and currents with a running window over one cycle of the specified frequency (port Freq).
      |  Input port "Sin_Cos" (a two-dimension signal) provides the reference frame required for the computation.
      |
      | input 1: must give the frequency of the fundamental (Hz)
      | Input 2: must contain a  [sin(wt)  cos(wt)] two dimension signal , where w is the rotation speed (rad/s) of the reference frame used for the computation..
      | input 3: Vectorized 3-phase  instantaneous voltage (Vabc)
      | input 4: Vectorized 3-phase instantaneous current (Iabc)
      |
      | Output 1: Vector [Mag_V Mag_I] of the fundamental values (Magnitude) of the voltage & current (peak values of the positive-sequence)
      | Output 2: 3-phase PQ measurement vector [P(W) Q (var)] evaluated at the specified frequency. Current flowing into an RL circuit will produce  positive active and reactive powers.
      |
      | For the first cycle of simulation, the ouputs are held constant using the values specified by the parameters "Initial input".
      | he value of the parameter "Minimum frequency" is used to determine the buffer size of the "Variable Transport Delay" block found inside this subsystem.
  Discrete 3-phase Positive-Sequence Fundamental Value : Subsystem  mask(Discrete 3-phase Positive-sequence fundamental value){Freq=60, Par_Init=[0 0], Ts=50e-6}
      mask prompts: Freq "Fundamental frequency (Hz):"; Par_Init "Initial input (positive component): [ Mag  Phase(degrees) ]"; Ts "Sample time:"
      mask help:
      | For a given fundamental frequency, this discrete block computes  the positive-sequence component (Magnitude and Phase)  of a set of three balanced or unbalanced signals which may contain harmonics. First and second outputs return respectively the magnitude and phase (degrees) of the fundamental.
      | For the first cycle of simulation, the ouputs are held constant to the values specified by the parameter "Initial input".
      mask init:
      | SamplesPerCycle=1/Freq/Ts;
      | RoundSamplesPerCycle=round(SamplesPerCycle);
      | Delay=RoundSamplesPerCycle*Ts - Ts/2;
      | Correction=SamplesPerCycle/RoundSamplesPerCycle - 1;
      | Real_Init=Par_Init(1)*cos(pi/180*Par_Init(2));
      | Imag_Init=Par_Init(1)*sin(pi/180*Par_Init(2));
  Discrete 3-phase Sequence Analyzer : Subsystem  mask(Discrete 3-Phase Sequence Analyzer){Freq=60, n=1, seq=Positive, Par_Init=[0 0], Ts=50e-6}
      mask prompts: Freq "Fundamental frequency (Hz):"; n "Harmonic n (0=DC; 1=fundamental) :"; seq "Sequence :"; Par_Init "Initial Input Pos. Seq. [Mag Phase(degrees)]:"; Ts "Sample time:"
      mask help:
      | This discrete block outputs the positive-,  negative-, zero- or all sequence component(s) (Magnitude and Phase)  of a set of three balanced or unbalanced signals  which may contain harmonics. The three sequence components are computed as folllows:
      |
      | V1 = 1/3 * (Va + a*Vb  + a^2 *Vc )
      | V2 = 1/3 * (Va + a ^2*Vb  +  a *Vc )
      | V0 = 1/3 * (Va +  Vb  +  Vc )
      | where: Va, Vb, Vc = input phasors at specified frequency
      |            a =exp(j *2pi/3) = 1 < + 120 deg.  complex operator
      |
      | The input contains the vectorized signal of the three [Va Vb Vc] sinusoidal signals
      | Output one and two give respectively the magnitude (peak value) and phase (degrees) of the specified sequence component(s).
      | For the first cycle of simulation, the ouputs are held constant to the values specified by the parameter "Initial input".
      mask init:
      | Pha20_On=0;
      | Mag_Init=Par_Init(1); Phase_Init=Par_Init(2);
      | k=2-(n==0);
      | a=exp(j*2*pi/3);
      | a2=exp(-j*2*pi/3);
      | switch seq
      | case 1,  % Pos. seq.
      |      PosOn=1;NegOn=0;ZeroOn=0;SelectElement=1;
      | case 2,  % Neg. seq.
      |      PosOn=0;NegOn=1;ZeroOn=0;SelectElement=2;
      | case 3,  % Zero. seq.
      |      PosOn=0;NegOn=0;ZeroOn=1;SelectElement=3;
      | case 4,  % All sequences
      |      PosOn=1;NegOn=1;ZeroOn=1;SelectElement=[1,2,3];Pha20_On=1;
      | end
      mask Help: A Fourier analysis over a sliding window of one cycle of the specified frequency is first applied on the three input signals to find phasors  Va, Vb and Vc at fundamental or harmonic  frequency . Then, the abc to 120  transformation is applied to obtain the positive-sequence V1, negative-sequence V2 and zero-sequence V0. You can use this block in a control system to measure a positive sequence voltage or current. It is not sensitive to harmonics otr unbalances. However, as  any filtered system, it introduces some delay. For example, its response to a step change of V1 is a one cycle ramp.
      mask StyleString: edit,edit,popup(Positive|Negative|Zero|Positive Negative Zero),edit,edit
  Discrete 3-phase Total Power : Subsystem  mask(Discrete 3-phase Total Power ){Freq=60, Par_Vinit=[0 0], Par_Iinit=[0 0], Ts=50e-6}
      mask prompts: Freq "Fundamental frequency (Hz):"; Par_Vinit "Voltage initial input: [ Mag  Phase(degrees) ]"; Par_Iinit "Current initial input: [ Mag  Phase(degrees) ]"; Ts "Sample time:"
      mask help:
      | This discrete block measures the 3-phase active power P associated with a periodic set of 3-phase voltages and currents which may contain harmonics. P is obtained by averaging the instantaneous power with a running window over one cycle of the fundamental frequency.
      |
      | input 1: Vectorized 3-phase  instantaneous voltage (Vabc)
      | input 2: Vectorized 3-phase instantaneous current (Iabc)
      |
      | Output : 3-phase active power. Current flowing into an RL circuit will produce  positive active power.
      |
      | For the first cycle of simulation, the ouput is held constant based on the values specified by the parameters "Initial input".
      mask init:
      | P_Init=3/2*Par_Vinit(1)*Par_Iinit(1)*cos(pi/180*(Par_Vinit(2)-Par_Iinit(2)));
  Discrete 3-phase  Positive-Sequence  Active & Reactive Power : Subsystem  mask(Discrete 3-phase Positive-Sequence Active & Reactive Power ){Freq=60, Par_Vinit=[0 0], Par_Iinit=[0 0], Ts=50e-6}
      mask prompts: Freq "Fundamental frequency (Hz):"; Par_Vinit "Voltage initial input: [ Mag  Phase(degrees) ]"; Par_Iinit "Current initial input: [ Mag  Phase(degrees) ]"; Ts "Sample time:"
      mask help:
      | This discrete block measures the 3-phase active power P and reactive power Q  associated with a periodic set of 3-phase voltages and currents which may contain harmonics. P and Q are calculated by evaluating the fundamental values (positive-sequence) of the input voltages and currents with a running window over one cycle of the fundamental frequency.
      |
      | input 1: Vectorized 3-phase  instantaneous voltage (Vabc)
      | input 2: Vectorized 3-phase instantaneous current (Iabc)
      |
      | Output 1: Vector [Mag_V Mag_I] of the fundamental values (Magnitude) of the voltage & current (peak values of the positive-sequence)
      | Output 2: 3-phase PQ measurement vector [P(W) Q (var)] evaluated at the fundamental frequency. Current flowing into an RL circuit will produce  positive active and reactive powers.
      |
      | For the first cycle of simulation, the ouputs are held constant using the values specified by the parameters "Initial input".
  FFT : Subsystem  mask(Fast Fourier Transform){Nsig=3, f1=50, Ts=500e-6, TsFFT=0.1, base=[1 1  1   ], nDec=0, mask=[1 -1  1  ], figure_N=2}
      mask prompts: Nsig "Input signal dimension Nsig:"; f1 "Fundamental frequency f1 (Hz):"; Ts "Sampling time Ts (s):"; TsFFT "FFT Sampling time F(n)"; base "Base peak value (1 for absolute , size=[1 Nsig ])"; nDec "Decimals to display RMS values on spectrum (0 for no text)"; mask "Mask (nomally ones(1,Nsig))"; figure_N "Figure number"
      mask help:
      | This block  implements FFT analysis  of  a vector of signals (dimension Nsig)  connected to input f(k).
      |
      | It can be used as a "real time" analyzer during simulation (note speed reduction !) or off-line by reading the signals from workspace after simulation.
      |
      | The F(n) output is a [Nh,Nsig] matrix of the Nsig signal spectra  (harmonic orders 0 to Nh-1), where Nh his the number of harmonics computed  given by : Nh= 1/f1/Ts/2.
      | The RMS output is a [5,Nsig] matrix of 5 different RMS values of the  Nsig signals: Line 1=  Total RMS; 2=DC component; 3=RMS value of fundamental; 4= RMS value of harmonics; 6=Total  AC rms .
      |
      | The  Nsig spectra are displayed on specified Figure number. By selecting different Figure numbers multiple blocks can be used. The "Mask" parameter is a a vector (1,Nsig) of  multiplication factors that can be used to modify plot appearance.
      |
      | See power_fft demo.
      mask init:
      | Navg=fix((1/f1)/Ts);
      mask Display: color('blue');disp('FFT')
  abc_to_dq0 Transformation : powerlib_extras/Measurements/abc_to_dq0 Transformation
  dq0-based Active & Reactive Power : powerlib_extras/Measurements/dq0-based Active & Reactive Power
  dq0_to_abc Transformation : powerlib_extras/Measurements/dq0_to_abc Transformation
